simulink model "Path_Planning"  (Simulink 8.3)
settings: Solver=ode5  StartTime=0.0  StopTime=120  FixedStep=0.01  RelTol=1e-3
values from neighbouring files (symbols this model uses):
  accuratepath = interplotation(path)    [Pathplanning.m]    (also in interplotation.m = [accuratepath;interp1([1,insertnum+2],[pathfromstartpoint(i,)
  d = 0.235    [Pathplanning.m]    (also in head.m)
libraries: simulink x1
settings Model: Creator=WXY  LastModifiedBy=WXY
settings DataIOCC: SignalLoggingSaveFormat=Dataset
settings DebuggingCC: UnderspecifiedInitializationDetection=Simplified  StateNameClashWarn=none
settings GRTTargetCC: CombineOutputUpdateFcns=on  GRTInterface=off

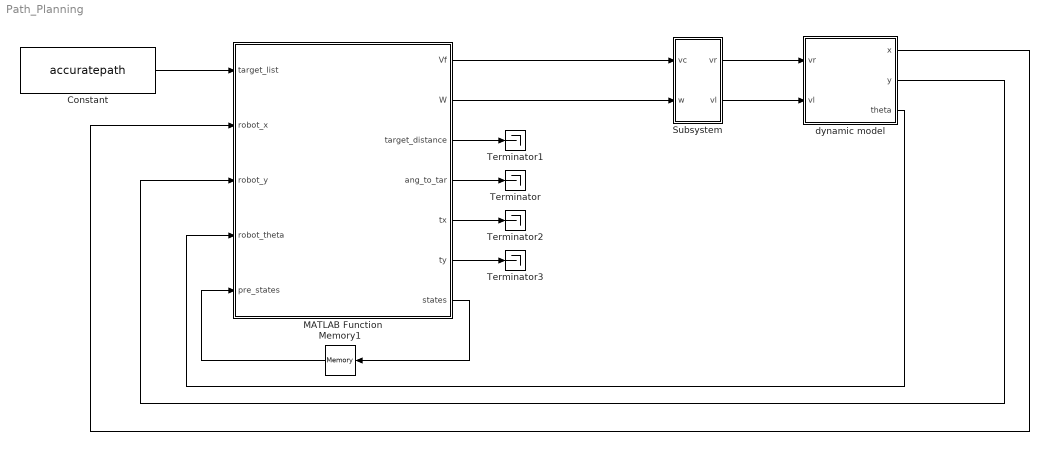
== system Path_Planning ==
  Constant : Constant  Value=accuratepath
  MATLAB Function : MATLAB Function  TreatAsAtomicUnit=on
  Memory1 : Memory  X0=[1]
  Subsystem : Subsystem
  Terminator{,1..3} (4 alike) : Terminator
  dynamic model : Subsystem
  wires:
  MATLAB Function/7(states) -> Memory1/1
  MATLAB Function/3(target_distance) -> Terminator1/1
  MATLAB Function/4(ang_to_tar) -> Terminator/1
  MATLAB Function/5(tx) -> Terminator2/1
  Subsystem/1(vr) -> dynamic model/1(vr)
  Subsystem/2(vl) -> dynamic model/2(vl)
  Constant/1 -> MATLAB Function/1(target_list)
  dynamic model/2(y) -> MATLAB Function/3(robot_y)
  dynamic model/1(x) -> MATLAB Function/2(robot_x)
  dynamic model/3(theta) -> MATLAB Function/4(robot_theta)
  MATLAB Function/1(Vf) -> Subsystem/1(vc)
  MATLAB Function/2(W) -> Subsystem/2(w)
  Memory1/1 -> MATLAB Function/5(pre_states)
  MATLAB Function/6(ty) -> Terminator3/1

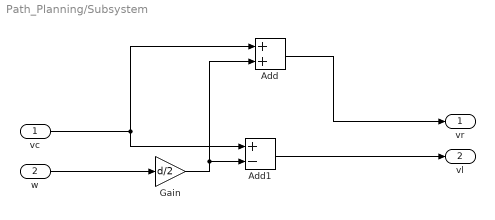
== system Path_Planning/Subsystem ==
  vc : Inport
  w : Inport  Port=2
  Add : Sum
  Add1 : Sum  Inputs=+-
  Gain : Gain  Gain=d/2
  vr : Outport
  vl : Outport  Port=2
  wires:
  vc/1 -> Add/1, Add1/1
  w/1 -> Gain/1
  Gain/1 -> Add/2, Add1/2
  Add/1 -> vr/1
  Add1/1 -> vl/1

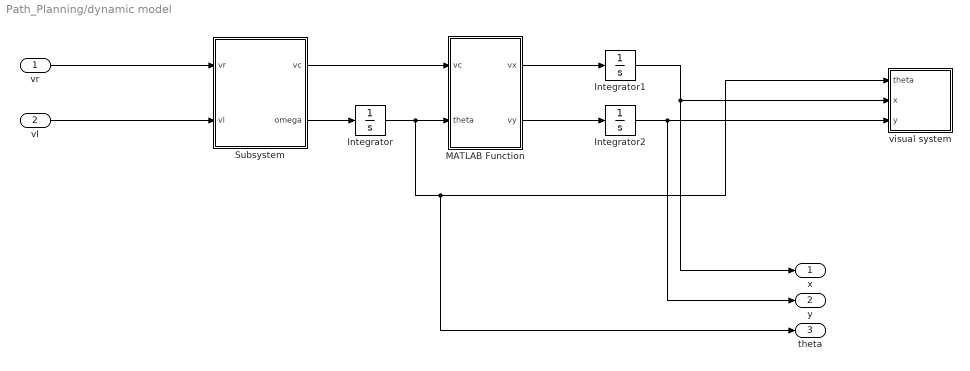
== system Path_Planning/dynamic model ==
  vr : Inport
  vl : Inport  Port=2
  Integrator : Integrator
  Integrator1 : Integrator
  Integrator2 : Integrator
  MATLAB Function : MATLAB Function  TreatAsAtomicUnit=on
  Subsystem : Subsystem
  visual system : Subsystem
  x : Outport
  y : Outport  Port=2
  theta : Outport  Port=3
  wires:
  MATLAB Function/2(vy) -> Integrator2/1
  MATLAB Function/1(vx) -> Integrator1/1
  vr/1 -> Subsystem/1(vr)
  vl/1 -> Subsystem/2(vl)
  Subsystem/1(vc) -> MATLAB Function/1(vc)
  Subsystem/2(omega) -> Integrator/1
  Integrator/1 -> theta/1, visual system/1(theta), MATLAB Function/2(theta)
  Integrator1/1 -> x/1, visual system/2(x)
  Integrator2/1 -> y/1, visual system/3(y)

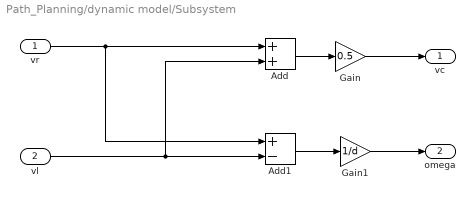
== system Path_Planning/dynamic model/Subsystem ==
  vr : Inport
  vl : Inport  Port=2
  Add : Sum
  Add1 : Sum  Inputs=+-
  Gain : Gain  Gain=0.5
  Gain1 : Gain  Gain=1/d
  vc : Outport
  omega : Outport  Port=2
  wires:
  vl/1 -> Add1/2, Add/2
  Gain/1 -> vc/1
  Add1/1 -> Gain1/1
  Add/1 -> Gain/1
  Gain1/1 -> omega/1
  vr/1 -> Add1/1, Add/1

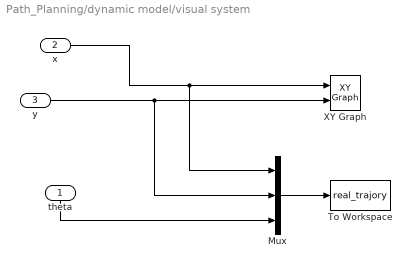
== system Path_Planning/dynamic model/visual system ==
  theta : Inport
  x : Inport  Port=2
  y : Inport  Port=3
  Mux : Mux  Inputs=3
  To Workspace : ToWorkspace  VariableName=real_trajory  SaveFormat=Structure With Time  SampleTime=-1
  XY Graph : simulink/Sinks/XY Graph  xmin=-1  xmax=10  ymin=-1  ymax=10  st=-1
  wires:
  Mux/1 -> To Workspace/1
  theta/1 -> Mux/3
  x/1 -> Mux/1, XY Graph/1
  y/1 -> Mux/2, XY Graph/2

== matlab function MATLAB Function ==
  data: target_list input double; Vf output double; robot_x input double; robot_y input double; robot_theta input double; pre_states input double; W output double; target_distance output double; ang_to_tar output double; tx output double; ty output double; states output double
function [Vf, W, target_distance, ang_to_tar, tx, ty, states] = ...
    WaypointControl(target_list, robot_x,robot_y,robot_theta, pre_states)
vlimit = 0.5; %最大限速
dist_thr = 0.1;
ang_thr = 10*pi/180;
method = 1;
step=1;
%step = 3; % 预估目标点的间隔
stop = 10;

%%%只需要改Kv_1 Kw_1就好
Kv_1 = 2; % 左轮速度常数   目标v=kv*x
Kw_1 = 1; % 左轮转角速度常数  目标w=kw*x

Kv_2 = 0.2;
Kw_2 = 0.9;
Psi_d = pi; % 机器人最终停止时角度（朝向）

% 初始化输出参数
 Vf=0;
 W=0;
 target_distance=0;
 ang_to_tar=0;
 finished_path_flag=0; 
 
 persistent Vf_1 end_flag;
 
 if isempty(Vf_1)
     Vf_1=0;
 end
 if isempty(end_flag)
    end_flag = 0;
 end
 
 %储存上一次的状态信息
states = pre_states;

rx =robot_x;
ry = robot_y;
rtheta = check_angle(robot_theta); %限定转角在 [-pi ,pi]之间


target_xy = [rx ry];  %当前坐标x y
[n xy] = size(target_list);  % n代表有n个点; xy=2
if n==2 && xy==1
    target_xy = [target_list(1,1) target_list(2,1)];
    n = 1;
else
    for i=1:n  %遍历所有规划的点
        if states(1) == i  %找到前面的规划点
            for j=1:xy
                if i < n-stop  %预瞄
                    target_xy(j) = target_list(i+stop, j);
                else
                    target_xy(j) = target_list(i, j);
                end
            end
        end
    end
end

tx = target_xy(1);
ty = target_xy(2);
target_distance = find_dist(rx, ry, tx, ty);
ang_to_tar= find_theta(rx, ry, rtheta, tx, ty);

if ((states(1) == n) && (target_distance <= dist_thr))  %到达终点或离终点

        Vf=0;
        W=0;
        
       if (end_flag == 1) && (target_distance <= dist_thr) % 最终到达目的地时朝向转到要求位置
            [Vf, W] = ClosedLoop_Sequential(0, check_angle(check_angle(Psi_d)-check_angle(rtheta)), vlimit, ang_thr, dist_thr, Kv_1, Kw_1, Vf_1); 
             Vf_1=Vf;
       end
   
else
    % 已经到达了目标点附近
    if (target_distance <= dist_thr) && (end_flag==0)
            states(1) = pre_states(1) + step;%1;
          if( pre_states(1) > 0 )      
             while (abs((target_list(states(1),1))-(target_list(pre_states(1),1)))<2*dist_thr) && (abs((target_list(states(1),2))-(target_list(pre_states(1),2)))<2*dist_thr)
                 if (states(1)<=(n-step))
                     states(1) = states(1) + step;%1;
                 else
                     states(1)=n;
                 end
             end
          else
              states(1)=states(1)+step;
          end
     
          %防止数组越界
         if states(1) >= n 
            states(1) = n;
            end_flag=1;  %停车
         end

    else
        if method == 2
            [Vf, W] = ClosedLoop_Both(target_distance,  ang_to_tar, vlimit, Kv_2, Kw_2);    
        else
            [Vf, W] = ClosedLoop_Sequential(target_distance,  ang_to_tar, vlimit, ang_thr, dist_thr, Kv_1, Kw_1, Vf_1); 
            Vf_1=Vf;
        end       
    end
    
end

return;

% 认为机器人转角应在-180到180度之间
function [y] = check_angle(x)
y = x;
while ( x > pi || x < -pi)
    if x > pi
        y = x - 2*pi;
    else
        y = x + 2*pi;
    end
end
return;

% 目标点与当前点距离
function dist = find_dist(rx, ry, tx, ty)
dist = sqrt((rx-tx)^2 + (ry-ty)^2);
return;

% 机器人当前需要转过的角度
function [theta]= find_theta(rx, ry, rtheta, tx, ty)

X = tx - rx;
Y = ty - ry;
theta = atan2(Y, X);
theta = check_angle(check_angle(theta)-check_angle(rtheta));

return;

% 根据目标距离和转角算出机器人的前进速度和转角速度
function [Vf, W] = ClosedLoop_Both(dist, theta, vlimit, Kv,Kw)

d = 0.23;
vmax = vlimit;
wmax = (2*vmax);
W = Kw*theta;

Vf = Kv * dist;

w_sign = sign(W); % 保留转角符号
if abs(W) > wmax
    W = w_sign*wmax;
end
if abs(Vf)> vlimit
    Vf = sign(Vf)*vlimit;%%%%% Vf = abs(Vf)*vlimit;
end

return;

% 仅前进或仅转弯
function [Vf, W] = ClosedLoop_Sequential(dist, theta, vlimit, ang_thr, dist_thr, Kv, Kw, Vf_1)

d = 0.23;
vmax = vlimit;
wmax = (2*vmax);

if (((abs(theta) > ang_thr))  && (Vf_1<0.01)) || (abs(theta) > 5*ang_thr) 
        W=Kw*theta;
        Vf=0;
        if abs(W)> wmax
            W=sign(W)*wmax;
        end
else
        Vf=Kv*dist;
       
        if abs(Vf)>vlimit
            Vf=sign(Vf)*vlimit;
        end
        
        W=0;
        
end
return;

== matlab function dynamic model/MATLAB Function ==
  data: vc input double; vx output double; theta input double; vy output double
function [vx,vy] = fcn(vc,theta)
%#codegen

vx=vc*cos(theta);
vy=vc*sin(theta);

end
